simulink model "SIM_20161201"  (R2017a)
settings: Solver=ode3  StartTime=0.0  StopTime=5  FixedStep=0.01  RelTol=1e-3  EnableMultiTasking=on
libraries: simulink x2
settings Model: Creator=Think  LastModifiedBy=Think
settings DataIOCC: LimitDataPoints=on  SaveFormat=Array
settings OptimizationCC: LifeSpan=inf
settings DebuggingCC: SolverPrmCheckMsg=warning  SFUnexpectedBacktrackingDiag=warning  SFNoUnconditionalDefaultTransitionDiag=warning  SFExecutionAtInitializationDiag=none
settings HardwareCC: ProdBitPerPointer=32  ProdBitPerSizeT=32  ProdBitPerPtrDiffT=32  ProdLargestAtomicFloat=None  ProdIntDivRoundTo=Undefined  ProdEndianess=Unspecified  ProdWordSize=32  ProdHWDeviceType=32-bit Generic
settings ModelReferenceCC: PropagateSignalLabelsOutOfModel=off
settings GRTTargetCC: TargetLangStandard=C89/C90 (ANSI)  GeneratePreprocessorConditionals=Disable all
settings ConfigComp: CovMetricSettings=dw  CovHtmlReporting=on  CovSaveCumulativeToWorkspaceVar=on  CovSaveSingleToWorkspaceVar=on  CovExternalEMLEnable=off  CovSFcnEnable=off

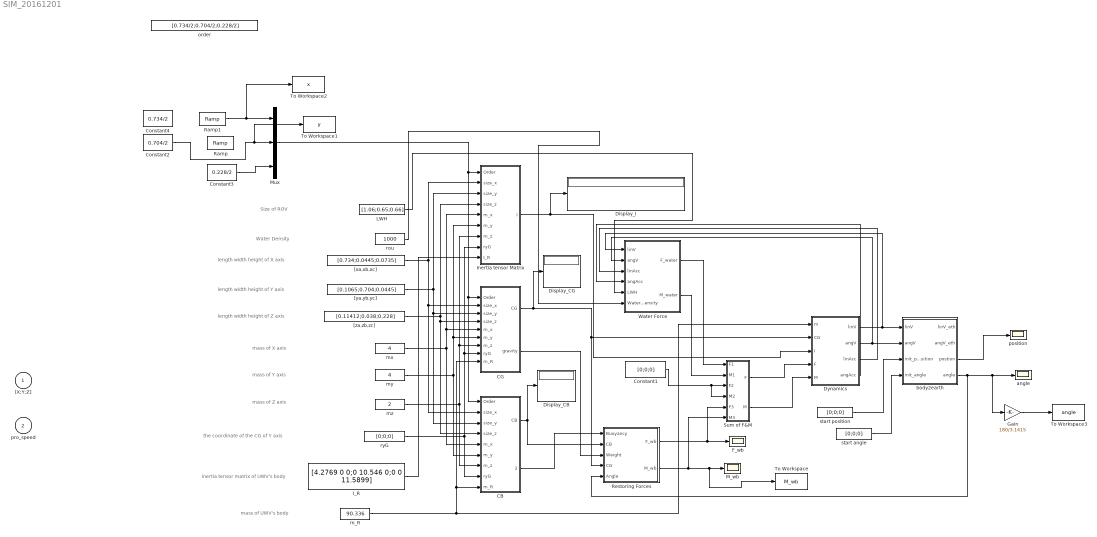
== system SIM_20161201 ==
  note: inertia tensor matrix of UWV's body
  note: mass of UWV's body
  note: length width height of X axis
  note: length width height of Y axis
  note: length width height of Z axis
  note: mass of X axis
  note: mass of Y axis
  note: mass of Z axis
  note: Water Density
  note: Size of ROV
  note: the coordinate of the CG of Y axis
  "[X;Y;Z]" : Inport
  pro_speed : Inport  Port=2
  CB : Subsystem
  CG : Subsystem
  Constant1 : Constant  Value=[0;0;0]
  Constant2 : Constant  Value=0.704/2
  Constant3 : Constant  Value=0.228/2
  Constant4 : Constant  Value=0.734/2
  Display_CB : Display
  Display_CG : Display
  Display_I : Display
  Dynamics : Subsystem
  F_wb : Scope
  Gain : Gain  Gain=180/3.1415
  I_R : Constant  Value=[4.2769 0 0;0 10.546 0;0 0 11.5899]
  Inertia tensor Matrix : Subsystem
  LWH : Constant  Value=[1.06;0.65;0.66]
  M_wb : Scope
  Mux : Mux  Inputs=3
  Ramp : simulink/Sources/Ramp  slope=0.0704  start=0  X0=0.704/2
  Ramp1 : simulink/Sources/Ramp  slope=0.0734  start=0  X0=0.734/2
  Restoring Forces : Subsystem
  Sum of F&M : Subsystem
  To Workspace : ToWorkspace  VariableName=M_wb  SaveFormat=Timeseries  SampleTime=-1
  To Workspace1 : ToWorkspace  VariableName=y  SaveFormat=Timeseries  SampleTime=-1
  To Workspace2 : ToWorkspace  VariableName=x  SaveFormat=Timeseries  SampleTime=-1
  To Workspace3 : ToWorkspace  VariableName=angle  SaveFormat=Timeseries  SampleTime=-1
  Water Force : Subsystem
  "[xa,xb,xc]" : Constant  Value=[0.734;0.0445;0.0735]
  "[ya,yb,yc]" : Constant  Value=[0.1065;0.704;0.0445]
  "[za,zb,zc]" : Constant  Value=[0.11412;0.038;0.228]
  angle : Scope
  "body2earth " : Subsystem
  m_R : Constant  Value=90.336
  mx : Constant  Value=4
  my : Constant  Value=4
  mz : Constant  Value=2
  order : Constant  Value=[0.734/2;0.704/2;0.228/2]
  position : Scope
  rou : Constant  Value=1000
  ryG : Constant  Value=[0;0;0]
  start angle : Constant  Value=[0;0;0]
  start position : Constant  Value=[0;0;0]
  wires:
  Dynamics/1(linV) -> Water Force/1(linV), "body2earth "/1(linV)
  Dynamics/2(angV) -> Water Force/2(angV), "body2earth "/2(angV)
  Restoring Forces/1(F_wb) -> Sum of F&M/5(F3), F_wb/1
  Restoring Forces/2(M_wb) -> Sum of F&M/6(M3), To Workspace/1, M_wb/1
  start position/1 -> "body2earth "/3(init_position)
  start angle/1 -> "body2earth "/4(init_angle)
  "body2earth "/3(postion) -> position/1
  I_R/1 -> Inertia tensor Matrix/9(I_R)
  m_R/1 -> CG/9(m_R), CB/9(m_R), Dynamics/1(m)
  CG/1(CG) -> Display_CG/1, Dynamics/2(CG), Restoring Forces/4(CG)
  Sum of F&M/1(F) -> Dynamics/4(F)
  Sum of F&M/2(M) -> Dynamics/5(M)
  Mux/1 -> CG/1(Order), CB/1(Order), Inertia tensor Matrix/1(Order)
  "[ya,yb,yc]"/1 -> CB/3(size_y), CG/3(size_y), Inertia tensor Matrix/3(size_y)
  "[za,zb,zc]"/1 -> Inertia tensor Matrix/4(size_z), CB/4(size_z), CG/4(size_z)
  mx/1 -> CB/5(m_x), CG/5(m_x), Inertia tensor Matrix/5(m_x)
  my/1 -> CB/6(m_y), CG/6(m_y), Inertia tensor Matrix/6(m_y)
  mz/1 -> CB/7(m_z), CG/7(m_z), Inertia tensor Matrix/7(m_z)
  ryG/1 -> CB/8(ryG), CG/8(ryG), Inertia tensor Matrix/8(ryG)
  "[xa,xb,xc]"/1 -> CB/2(size_x), CG/2(size_x), Inertia tensor Matrix/2(size_x)
  CB/1(CB) -> Restoring Forces/2(CB), Display_CB/1
  Inertia tensor Matrix/1(I) -> Display_I/1, Dynamics/3(I)
  CB/2(Buoyancy) -> Restoring Forces/1(Buoyancy)
  CG/2(gravity) -> Restoring Forces/3(Weight)
  Constant1/1 -> Sum of F&M/4(M2), Sum of F&M/3(F2)
  Constant3/1 -> Mux/3
  Constant2/1 -> Mux/2, To Workspace1/1
  Ramp1/1 -> To Workspace2/1, Mux/1
  Gain/1 -> To Workspace3/1
  "body2earth "/4(angle) -> Restoring Forces/5(Angle), Gain/1, angle/1
  Water Force/1(F_water) -> Sum of F&M/1(F1)
  Water Force/2(M_water) -> Sum of F&M/2(M1)
  Dynamics/3(linAcc) -> Water Force/3(linAcc)
  Dynamics/4(angAcc) -> Water Force/4(angAcc)
  LWH/1 -> Water Force/5(LWH)
  rou/1 -> Water Force/6(WaterDensity)

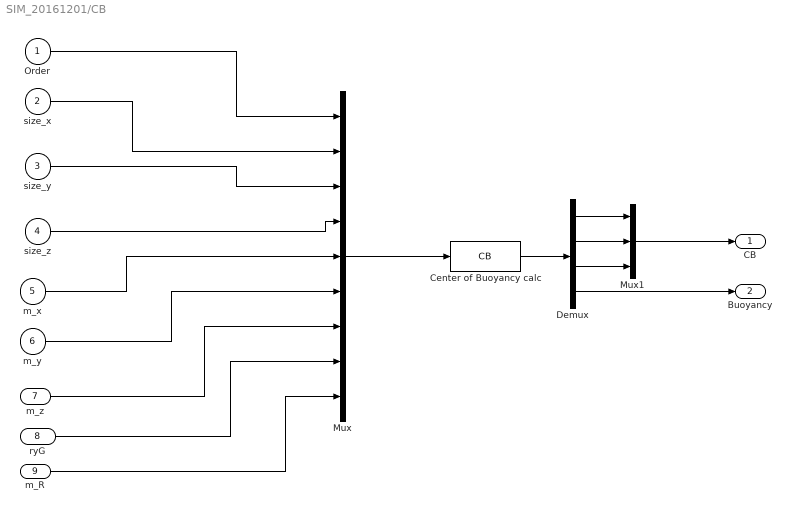
== system SIM_20161201/CB ==
  Order : Inport
  size_x : Inport  Port=2
  size_y : Inport  Port=3
  size_z : Inport  Port=4
  m_x : Inport  Port=5
  m_y : Inport  Port=6
  m_z : Inport  Port=7
  ryG : Inport  Port=8
  m_R : Inport  Port=9
  Center of Buoyancy calc : MATLABFcn  MATLABFcn=CB  Output1D=off
  Demux : Demux
  Mux : Mux  Inputs=9
  Mux1 : Mux  Inputs=3
  CB : Outport
  Buoyancy : Outport  Port=2
  wires:
  m_x/1 -> Mux/5
  m_y/1 -> Mux/6
  size_x/1 -> Mux/2
  ryG/1 -> Mux/8
  size_z/1 -> Mux/4
  Order/1 -> Mux/1
  size_y/1 -> Mux/3
  m_R/1 -> Mux/9
  m_z/1 -> Mux/7
  Mux/1 -> Center of Buoyancy calc/1
  Center of Buoyancy calc/1 -> Demux/1
  Demux/1 -> Mux1/1
  Demux/2 -> Mux1/2
  Demux/3 -> Mux1/3
  Demux/4 -> Buoyancy/1
  Mux1/1 -> CB/1

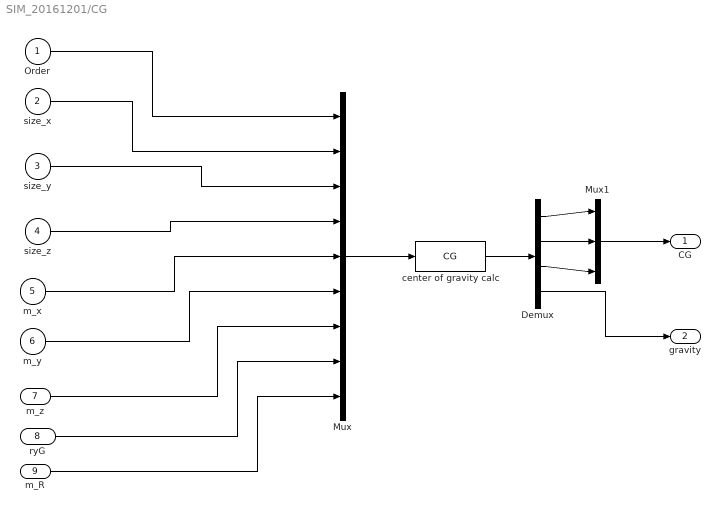
== system SIM_20161201/CG ==
  Order : Inport
  size_x : Inport  Port=2
  size_y : Inport  Port=3
  size_z : Inport  Port=4
  m_x : Inport  Port=5
  m_y : Inport  Port=6
  m_z : Inport  Port=7
  ryG : Inport  Port=8
  m_R : Inport  Port=9
  Demux : Demux
  Mux : Mux  Inputs=9
  Mux1 : Mux  Inputs=3
  center of gravity calc : MATLABFcn  MATLABFcn=CG  Output1D=off
  CG : Outport
  gravity : Outport  Port=2
  wires:
  m_R/1 -> Mux/9
  Mux/1 -> center of gravity calc/1
  ryG/1 -> Mux/8
  Order/1 -> Mux/1
  m_z/1 -> Mux/7
  size_y/1 -> Mux/3
  size_z/1 -> Mux/4
  m_x/1 -> Mux/5
  size_x/1 -> Mux/2
  m_y/1 -> Mux/6
  center of gravity calc/1 -> Demux/1
  Demux/1 -> Mux1/1
  Demux/2 -> Mux1/2
  Demux/3 -> Mux1/3
  Mux1/1 -> CG/1
  Demux/4 -> gravity/1

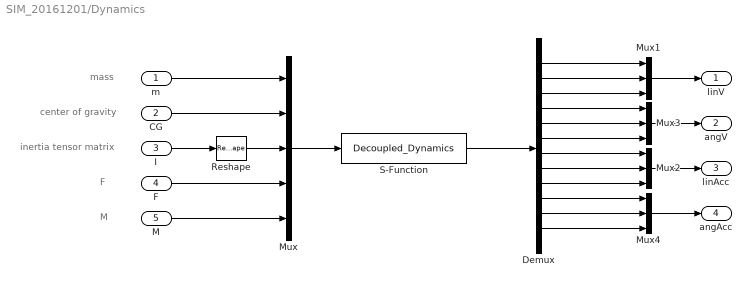
== system SIM_20161201/Dynamics ==
  note: inertia tensor matrix
  note: F
  note: center of gravity
  note: mass
  note: M
  m : Inport
  CG : Inport  Port=2
  I : Inport  Port=3
  F : Inport  Port=4
  M : Inport  Port=5
  Demux : Demux  Outputs=12
  Mux : Mux  Inputs=5
  Mux{1..4} (4 alike) : Mux  Inputs=3
  Reshape : Reshape
  S-Function : S-Function  FunctionName=Decoupled_Dynamics  SFunctionDeploymentMode=off  EnableBusSupport=off
  linV : Outport
  angV : Outport  Port=2
  linAcc : Outport  Port=3
  angAcc : Outport  Port=4
  wires:
  CG/1 -> Mux/2
  I/1 -> Reshape/1
  m/1 -> Mux/1
  Reshape/1 -> Mux/3
  F/1 -> Mux/4
  Mux/1 -> S-Function/1
  S-Function/1 -> Demux/1
  Demux/1 -> Mux1/1
  Demux/2 -> Mux1/2
  Demux/3 -> Mux1/3
  Demux/4 -> Mux3/1
  Demux/5 -> Mux3/2
  Demux/6 -> Mux3/3
  Mux1/1 -> linV/1
  Demux/7 -> Mux2/1
  Demux/8 -> Mux2/2
  Demux/9 -> Mux2/3
  Demux/10 -> Mux4/1
  Demux/11 -> Mux4/2
  Demux/12 -> Mux4/3
  Mux2/1 -> linAcc/1
  Mux3/1 -> angV/1
  Mux4/1 -> angAcc/1
  M/1 -> Mux/5

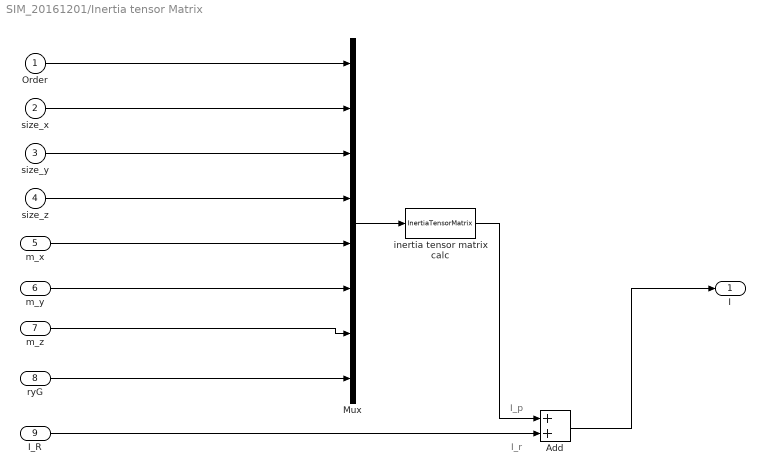
== system SIM_20161201/Inertia tensor Matrix ==
  note: I_r
  note: I_p
  Order : Inport
  size_x : Inport  Port=2
  size_y : Inport  Port=3
  size_z : Inport  Port=4
  m_x : Inport  Port=5
  m_y : Inport  Port=6
  m_z : Inport  Port=7
  ryG : Inport  Port=8
  I_R : Inport  Port=9
  Add : Sum
  Mux : Mux  Inputs=8
  inertia tensor matrix calc : MATLABFcn  MATLABFcn=InertiaTensorMatrix  Output1D=off
  I : Outport
  wires:
  inertia tensor matrix calc/1 -> Add/1
  I_R/1 -> Add/2
  Mux/1 -> inertia tensor matrix calc/1
  m_z/1 -> Mux/7
  size_z/1 -> Mux/4
  m_x/1 -> Mux/5
  Order/1 -> Mux/1
  m_y/1 -> Mux/6
  size_x/1 -> Mux/2
  size_y/1 -> Mux/3
  ryG/1 -> Mux/8
  Add/1 -> I/1

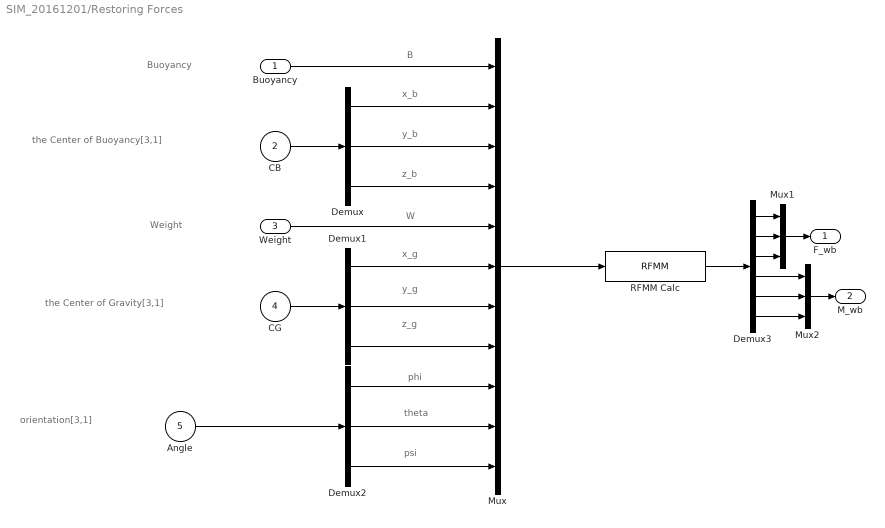
== system SIM_20161201/Restoring Forces ==
  note: psi
  note: theta
  note: phi
  note: W
  note: x_b
  note: B
  note: Buoyancy
  note: the Center of Buoyancy[3,1]
  note: Weight
  note: the Center of Gravity[3,1]
  note: orientation[3,1]
  note: y_b
  note: z_b
  note: x_g
  note: y_g
  note: z_g
  Buoyancy : Inport
  CB : Inport  Port=2
  Weight : Inport  Port=3
  CG : Inport  Port=4
  Angle : Inport  Port=5
  Demux : Demux  Outputs=3
  Demux1 : Demux  Outputs=3
  Demux2 : Demux  Outputs=3
  Demux3 : Demux  Outputs=6
  Mux : Mux  Inputs=11
  Mux1 : Mux  Inputs=3
  Mux2 : Mux  Inputs=3
  RFMM Calc : MATLABFcn  MATLABFcn=RFMM  OutputDimensions=6
  F_wb : Outport
  M_wb : Outport  Port=2
  wires:
  CB/1 -> Demux/1
  CG/1 -> Demux1/1
  Buoyancy/1 -> Mux/1
  Demux/1 -> Mux/2
  Demux/2 -> Mux/3
  Demux/3 -> Mux/4
  Weight/1 -> Mux/5
  Demux1/1 -> Mux/6
  Demux1/2 -> Mux/7
  Demux1/3 -> Mux/8
  Demux2/1 -> Mux/9
  Demux2/2 -> Mux/10
  Demux2/3 -> Mux/11
  Mux/1 -> RFMM Calc/1
  Angle/1 -> Demux2/1
  Demux3/6 -> Mux2/3
  Demux3/4 -> Mux2/1
  Demux3/5 -> Mux2/2
  Mux2/1 -> M_wb/1
  Demux3/3 -> Mux1/3
  Demux3/1 -> Mux1/1
  Demux3/2 -> Mux1/2
  Mux1/1 -> F_wb/1
  RFMM Calc/1 -> Demux3/1

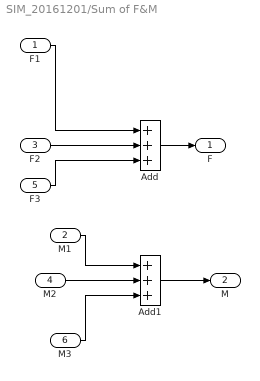
== system SIM_20161201/Sum of F&M ==
  F1 : Inport
  M1 : Inport  Port=2
  F2 : Inport  Port=3
  M2 : Inport  Port=4
  F3 : Inport  Port=5
  M3 : Inport  Port=6
  Add : Sum  Inputs=+++
  Add1 : Sum  Inputs=+++
  F : Outport
  M : Outport  Port=2
  wires:
  F1/1 -> Add/1
  F2/1 -> Add/2
  Add/1 -> F/1
  F3/1 -> Add/3
  M1/1 -> Add1/1
  M2/1 -> Add1/2
  Add1/1 -> M/1
  M3/1 -> Add1/3

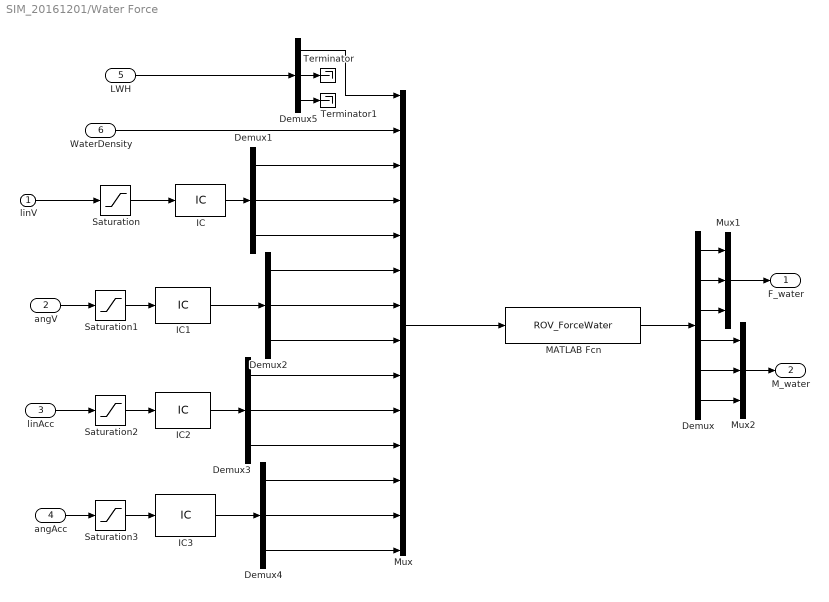
== system SIM_20161201/Water Force ==
  linV : Inport
  angV : Inport  Port=2
  linAcc : Inport  Port=3
  angAcc : Inport  Port=4
  LWH : Inport  Port=5
  WaterDensity : Inport  Port=6
  Demux : Demux  Outputs=6
  Demux{1..5} (5 alike) : Demux  Outputs=3
  IC{,1..3} (4 alike) : InitialCondition  Value=0.001
  MATLAB Fcn : MATLABFcn  MATLABFcn=ROV_ForceWater  OutputDimensions=6  Output1D=off
  Mux : Mux  Inputs=14
  Mux1 : Mux  Inputs=3
  Mux2 : Mux  Inputs=3
  Saturation : Saturate  UpperLimit=0.3  LowerLimit=-0.3
  Saturation1 : Saturate  UpperLimit=0.4  LowerLimit=-0.4
  Saturation2 : Saturate  UpperLimit=2.5  LowerLimit=-2.5
  Saturation3 : Saturate  UpperLimit=10  LowerLimit=-10
  Terminator : Terminator
  Terminator1 : Terminator
  F_water : Outport
  M_water : Outport  Port=2
  wires:
  Demux4/3 -> Mux/14
  Demux4/2 -> Mux/13
  Demux4/1 -> Mux/12
  Demux3/3 -> Mux/11
  Demux3/2 -> Mux/10
  Demux3/1 -> Mux/9
  Demux2/3 -> Mux/8
  Demux2/2 -> Mux/7
  Demux2/1 -> Mux/6
  Demux1/3 -> Mux/5
  Demux1/1 -> Mux/3
  Demux1/2 -> Mux/4
  Mux2/1 -> M_water/1
  Demux/4 -> Mux2/1
  Demux/6 -> Mux2/3
  Demux/5 -> Mux2/2
  Mux1/1 -> F_water/1
  Demux/1 -> Mux1/1
  Demux/3 -> Mux1/3
  Demux/2 -> Mux1/2
  MATLAB Fcn/1 -> Demux/1
  Mux/1 -> MATLAB Fcn/1
  WaterDensity/1 -> Mux/2
  LWH/1 -> Demux5/1
  Demux5/1 -> Mux/1
  Demux5/2 -> Terminator/1
  Demux5/3 -> Terminator1/1
  linV/1 -> Saturation/1
  angV/1 -> Saturation1/1
  linAcc/1 -> Saturation2/1
  angAcc/1 -> Saturation3/1
  IC/1 -> Demux1/1
  IC1/1 -> Demux2/1
  IC2/1 -> Demux3/1
  IC3/1 -> Demux4/1
  Saturation/1 -> IC/1
  Saturation1/1 -> IC1/1
  Saturation2/1 -> IC2/1
  Saturation3/1 -> IC3/1

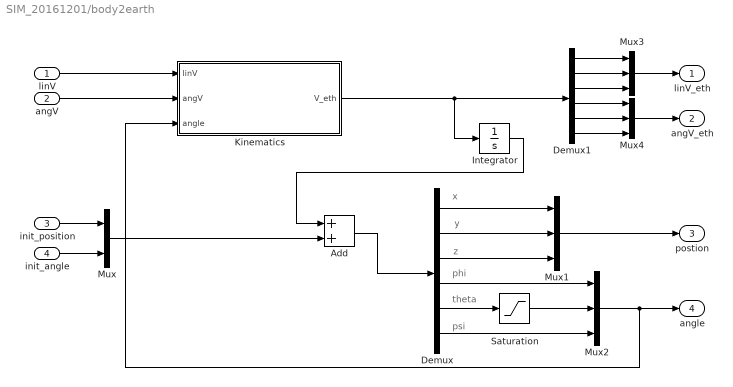
== system SIM_20161201/body2earth  ==
  note: psi
  note: theta
  note: phi
  note: z
  note: y
  note: x
  linV : Inport
  angV : Inport  Port=2
  init_position : Inport  Port=3
  init_angle : Inport  Port=4
  Add : Sum
  Demux : Demux  Outputs=6
  Demux1 : Demux  Outputs=6
  Integrator : Integrator
  Kinematics : Subsystem
  Mux : Mux  Inputs=2
  Mux{1..4} (4 alike) : Mux  Inputs=3
  Saturation : Saturate  UpperLimit=1.4  LowerLimit=-1.4
  linV_eth : Outport
  angV_eth : Outport  Port=2
  postion : Outport  Port=3
  angle : Outport  Port=4
  wires:
  Integrator/1 -> Add/1
  Add/1 -> Demux/1
  Demux/1 -> Mux1/1
  Demux/2 -> Mux1/2
  Demux/3 -> Mux1/3
  Demux/5 -> Saturation/1
  Saturation/1 -> Mux2/2
  Mux1/1 -> postion/1
  Kinematics/1(V_eth) -> Integrator/1, Demux1/1
  linV/1 -> Kinematics/1(linV)
  Demux/4 -> Mux2/1
  Demux/6 -> Mux2/3
  Mux2/1 -> Kinematics/3(angle), angle/1
  init_angle/1 -> Mux/2
  init_position/1 -> Mux/1
  Mux/1 -> Add/2
  angV/1 -> Kinematics/2(angV)
  Mux3/1 -> linV_eth/1
  Demux1/6 -> Mux4/3
  Demux1/1 -> Mux3/1
  Demux1/2 -> Mux3/2
  Demux1/3 -> Mux3/3
  Demux1/4 -> Mux4/1
  Demux1/5 -> Mux4/2
  Mux4/1 -> angV_eth/1

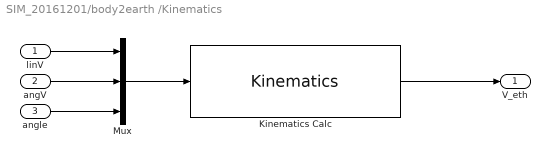
== system SIM_20161201/body2earth /Kinematics ==
  linV : Inport
  angV : Inport  Port=2
  angle : Inport  Port=3
  Kinematics Calc : MATLABFcn  MATLABFcn=Kinematics  OutputDimensions=6
  Mux : Mux  Inputs=3
  V_eth : Outport
  wires:
  linV/1 -> Mux/1
  Mux/1 -> Kinematics Calc/1
  angV/1 -> Mux/2
  angle/1 -> Mux/3
  Kinematics Calc/1 -> V_eth/1
